simulink model "ddc_bpm_476_066_hov"  (Simulink 7.8)
settings: Solver=ode45  StartTime=0.0  StopTime=2.56e-3  RelTol=1e-3
undefined symbols (not defined in the file): dt_sim, frev_476, Fs_adc, xlipgetpartsetting
libraries: xbsIndex_r4 x654, simulink x3
(part 3 of 7)

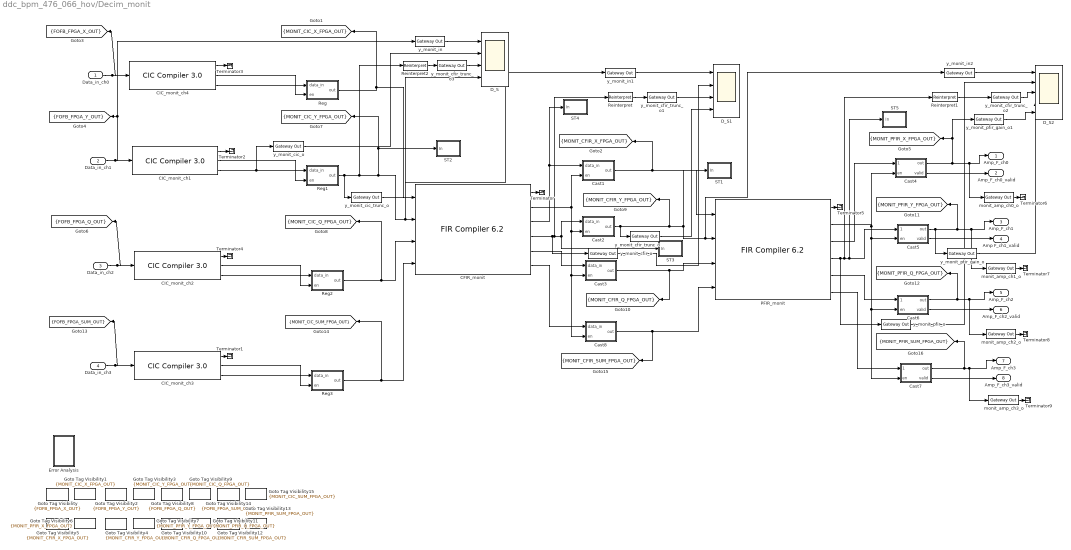
== system ddc_bpm_476_066_hov/Decim_monit ==
  Data_in_ch0 : Inport
  Data_in_ch1 : Inport  Port=2
  Data_in_ch2 : Inport  Port=3
  Data_in_ch3 : Inport  Port=4
  CFIR_monit : xbsIndex_r4/FIR Compiler 6.2   coefficientvector=hcfir_sec.Numerator  coefficient_sets=1  filter_type=Decimation  rate_change_type=Integer  interpolation_rate=1  decimation_rate=2  number_channels=1  ratespecification=Hardware_Oversampling_Rate  sampleperiod=5565000  hardwareoversamplingrate=1  filter_architecture=Systolic_Multiply_Accumulate  coefficient_reload=off  coefficient_sign=Signed  quantization=Quantize_Only  coefficient_width=16  bestprecision=on  coefficient_fractional_bits=15  coefficient_structure=Inferred  number_paths=4  output_rounding_mode=Convergent_Rounding_to_Even  output_width=25  optimization_goal=Area  data_has_tlast=Not_Required  m_data_has_tready=off  s_data_has_fifo=off  s_data_has_tuser=Not_Required  m_data_has_tuser=Not_Required  s_config_sync_mode=On_Vector  s_config_method=Single  num_reload_slots=1  has_aclken=off  has_aresetn=off  multi_column_support=Disabled  columnconfig='11'  inter_column_pipe_length=4  data_buffer_type=Automatic  coefficient_buffer_type=Automatic  input_buffer_type=Automatic  output_buffer_type=Automatic  preference_for_other_storage=Automatic  trim_axipin_name=on  passband_min=0.0  passband_max=0.5  stopband_min=0.5  stopband_max=1.0  filter_selection=1  gui_behaviour=Sysgen_GUI  data_sign=Signed  data_width=16  data_fractional_bits=0  wrapper_available=true  ip_wrap_arbitrary_binary_point=true  ip_name=FIR Compiler  ip_version=6.2  dsptool_ready=true  ipcore_usecache=true  ipcore_useipmodelcache=true  ipcore_xco_need_fpga_part=true  port_translation_map={ 'aclken' => 'en', 'aresetn' => 'rst' }  run_core_at_system_period=true  ipcore_fpga_part=xlipgetpartsetting(gcb, {'virtex6', 'xc6vlx75t', '-3', 'ff784'})  structural_sim=false  block_type=fir_compiler_v6_2
      settings: infoedit=Maximum Possible : Maximizes oversampling rate. Abstracted input handshake (no s_data_tvalid) and automatic rate propagation.<br>Hardware Oversampling Rate : Specifies oversampling rate relative to the input sample period. Abstracted input handshake (no s_data_tvalid) and automatic rate propagation.<br>Sample Period : Specifies absolute oversampling rate. No input handshake abstraction (exposes s_data_tvalid) and no rate propagation.
  CIC_monit_ch{1..4} (4 alike) : xbsIndex_r4/CIC Compiler 3.0   filter_type=Decimation  number_of_stages=5  differential_delay=2  number_of_channels=1  sample_rate_changes=Fixed  fixed_or_initial_rate=R_sec  minimum_rate=2500  maximum_rate=2500  ratespecification=Maximum_Possible  sampleperiod=1  hardwareoversamplingrate=1113  quantization=Truncation  output_data_width=25  use_xtreme_dsp_slice=off  use_streaming_interface=on  has_aclken=off  has_aresetn=off  has_dout_tready=off  trim_axipin_name=on  gui_behaviour=Sysgen_GUI  input_data_width=18  ip_name=CIC Compiler  ip_version=3.0  dsptool_ready=true  wrapper_available=true  port_translation_map={ 'aclken' => 'en', 'aresetn' => 'rst' }  ipcore_xco_need_fpga_part=true  ipcore_fpga_part=xlipgetpartsetting(gcb, {'virtex7', 'xc7v1500t', '-2', 'fhg1157'})  ipcore_verbose=false  block_type=cic_compiler_v3_0
  Cast1 : Subsystem
  Cast2 : Subsystem
  Cast3 : Subsystem
  Cast4 : Subsystem
  Cast5 : Subsystem
  Cast6 : Subsystem
  Cast7 : Subsystem
  Cast8 : Subsystem
  D_S : Scope  NumInputPorts=4
      settings: TimeRange=0.0004  YMin=0.0062~37100~0.00221125~0.0044225  YMax=0.00685~37140~0.00221375~0.0044275  MaxDataPoints=1000000  SampleInput=on
  D_S1 : Scope  NumInputPorts=4
      settings: TimeRange=0.0004  YMin=0.00442481~0.00443029~0.00443029~0.00446463  YMax=0.00442481~0.00443029~0.00443029~0.00446463  SaveName=ScopeData2  MaxDataPoints=1000000  SampleInput=on
  D_S2 : Scope  NumInputPorts=5
      settings: TimeRange=0.0004  YMin=0.00442791~-1~3.8147e-006~-3.33786e-006~-3.33786e-006  YMax=0.00442791~1~3.8147e-006~-3.33786e-006~-3.33786e-006  SaveName=ScopeData3  MaxDataPoints=1000000  SampleInput=on
  Error Analysis : Subsystem
  Goto Tag Visibility : GotoTagVisibility  GotoTag=FOFB_FPGA_X_OUT
  Goto Tag Visibility1 : GotoTagVisibility  GotoTag=MONIT_CIC_X_FPGA_OUT
  Goto Tag Visibility10 : GotoTagVisibility  GotoTag=MONIT_CFIR_Q_FPGA_OUT
  Goto Tag Visibility11 : GotoTagVisibility  GotoTag=MONIT_PFIR_Q_FPGA_OUT
  Goto Tag Visibility12 : GotoTagVisibility  GotoTag=MONIT_CFIR_SUM_FPGA_OUT
  Goto Tag Visibility13 : GotoTagVisibility  GotoTag=MONIT_PFIR_SUM_FPGA_OUT
  Goto Tag Visibility14 : GotoTagVisibility  GotoTag=FOFB_FPGA_SUM_OUT
  Goto Tag Visibility15 : GotoTagVisibility  GotoTag=MONIT_CIC_SUM_FPGA_OUT
  Goto Tag Visibility2 : GotoTagVisibility  GotoTag=FOFB_FPGA_Y_OUT
  Goto Tag Visibility3 : GotoTagVisibility  GotoTag=MONIT_CIC_Y_FPGA_OUT
  Goto Tag Visibility4 : GotoTagVisibility  GotoTag=MONIT_CFIR_Y_FPGA_OUT
  Goto Tag Visibility5 : GotoTagVisibility  GotoTag=MONIT_CFIR_X_FPGA_OUT
  Goto Tag Visibility6 : GotoTagVisibility  GotoTag=MONIT_PFIR_X_FPGA_OUT
  Goto Tag Visibility7 : GotoTagVisibility  GotoTag=MONIT_PFIR_Y_FPGA_OUT
  Goto Tag Visibility8 : GotoTagVisibility  GotoTag=FOFB_FPGA_Q_OUT
  Goto Tag Visibility9 : GotoTagVisibility  GotoTag=MONIT_CIC_Q_FPGA_OUT
  PFIR_monit : xbsIndex_r4/FIR Compiler 6.2   coefficientvector=hpfir_sec.Numerator  coefficient_sets=1  filter_type=Decimation  rate_change_type=Integer  interpolation_rate=1  decimation_rate=2  number_channels=1  ratespecification=Hardware_Oversampling_Rate  sampleperiod=5565000  hardwareoversamplingrate=1  filter_architecture=Systolic_Multiply_Accumulate  coefficient_reload=off  coefficient_sign=Signed  quantization=Quantize_Only  coefficient_width=16  bestprecision=on  coefficient_fractional_bits=15  coefficient_structure=Inferred  number_paths=4  output_rounding_mode=Convergent_Rounding_to_Even  output_width=25  optimization_goal=Area  data_has_tlast=Not_Required  m_data_has_tready=off  s_data_has_fifo=off  s_data_has_tuser=Not_Required  m_data_has_tuser=Not_Required  s_config_sync_mode=On_Vector  s_config_method=Single  num_reload_slots=1  has_aclken=off  has_aresetn=off  multi_column_support=Disabled  columnconfig='22'  inter_column_pipe_length=4  data_buffer_type=Automatic  coefficient_buffer_type=Automatic  input_buffer_type=Automatic  output_buffer_type=Automatic  preference_for_other_storage=Automatic  trim_axipin_name=on  passband_min=0.0  passband_max=0.5  stopband_min=0.5  stopband_max=1.0  filter_selection=1  gui_behaviour=Sysgen_GUI  data_sign=Signed  data_width=16  data_fractional_bits=0  wrapper_available=true  ip_wrap_arbitrary_binary_point=true  ip_name=FIR Compiler  ip_version=6.2  dsptool_ready=true  ipcore_usecache=true  ipcore_useipmodelcache=true  ipcore_xco_need_fpga_part=true  port_translation_map={ 'aclken' => 'en', 'aresetn' => 'rst' }  run_core_at_system_period=true  ipcore_fpga_part=xlipgetpartsetting(gcb, {'virtex6', 'xc6vlx75t', '-3', 'ff784'})  structural_sim=false  block_type=fir_compiler_v6_2
      settings: infoedit=Maximum Possible : Maximizes oversampling rate. Abstracted input handshake (no s_data_tvalid) and automatic rate propagation.<br>Hardware Oversampling Rate : Specifies oversampling rate relative to the input sample period. Abstracted input handshake (no s_data_tvalid) and automatic rate propagation.<br>Sample Period : Specifies absolute oversampling rate. No input handshake abstraction (exposes s_data_tvalid) and no rate propagation.
  Reg : Subsystem
  Reg1 : Subsystem
  Reg2 : Subsystem
  Reg3 : Subsystem
  Reinterpret : xbsIndex_r4/Reinterpret  force_arith_type=on  arith_type="Signed  (2's comp)"  force_bin_pt=off  bin_pt=41  block_type=cast
      settings: block_version=VER_STRING_GOES_HERE
  Reinterpret1 : xbsIndex_r4/Reinterpret  force_arith_type=on  arith_type="Signed  (2's comp)"  force_bin_pt=off  bin_pt=41  block_type=cast
      settings: block_version=VER_STRING_GOES_HERE
  Reinterpret2 : xbsIndex_r4/Reinterpret  force_arith_type=on  arith_type="Signed  (2's comp)"  force_bin_pt=on  bin_pt=23  block_type=cast
      settings: block_version=VER_STRING_GOES_HERE
  ST1 : Subsystem
  ST2 : Subsystem
  ST3 : Subsystem
  ST4 : Subsystem
  ST5 : Subsystem
  Terminator{,1..9} (10 alike) : Terminator
  monit_amp_ch0_o : xbsIndex_r4/Gateway Out  inherit_from_input=on  hdl_port=on  timing_constraint=Data Rate  locs_specified=off  LOCs={}  UseAsDAC=off  DACChannel='1'  block_type=gatewayout
      settings: infoedit="Gateway out block.  Converts Xilinx fixed-point or floating-point type inputs into ouputs of type Simulink integer, single, double, or fixed point.<br><br>Hardware notes:  In hardware these blocks become top level output ports or are discarded, depending on how they are configured."
  monit_amp_ch1_o : xbsIndex_r4/Gateway Out  inherit_from_input=on  hdl_port=on  timing_constraint=Data Rate  locs_specified=off  LOCs={}  UseAsDAC=off  DACChannel='1'  block_type=gatewayout
      settings: infoedit="Gateway out block.  Converts Xilinx fixed-point or floating-point type inputs into ouputs of type Simulink integer, single, double, or fixed point.<br><br>Hardware notes:  In hardware these blocks become top level output ports or are discarded, depending on how they are configured."
  monit_amp_ch2_o : xbsIndex_r4/Gateway Out  inherit_from_input=on  hdl_port=on  timing_constraint=Data Rate  locs_specified=off  LOCs={}  UseAsDAC=off  DACChannel='1'  block_type=gatewayout
      settings: infoedit="Gateway out block.  Converts Xilinx fixed-point or floating-point type inputs into ouputs of type Simulink integer, single, double, or fixed point.<br><br>Hardware notes:  In hardware these blocks become top level output ports or are discarded, depending on how they are configured."
  monit_amp_ch3_o : xbsIndex_r4/Gateway Out  inherit_from_input=on  hdl_port=on  timing_constraint=Data Rate  locs_specified=off  LOCs={}  UseAsDAC=off  DACChannel='1'  block_type=gatewayout
      settings: infoedit="Gateway out block.  Converts Xilinx fixed-point or floating-point type inputs into ouputs of type Simulink integer, single, double, or fixed point.<br><br>Hardware notes:  In hardware these blocks become top level output ports or are discarded, depending on how they are configured."
  y_monit_cfir_o : xbsIndex_r4/Gateway Out  inherit_from_input=on  hdl_port=off  timing_constraint=None  locs_specified=off  LOCs={}  UseAsDAC=off  DACChannel='1'  block_type=gatewayout
      settings: infoedit="Gateway out block.  Converts Xilinx fixed-point or floating-point type inputs into ouputs of type Simulink integer, single, double, or fixed point.<br><br>Hardware notes:  In hardware these blocks become top level output ports or are discarded, depending on how they are configured."
  y_monit_cfir_trunc_o{,1..3} (4 alike) : xbsIndex_r4/Gateway Out  inherit_from_input=on  hdl_port=off  timing_constraint=None  locs_specified=off  LOCs={}  UseAsDAC=off  DACChannel='1'  block_type=gatewayout
      settings: infoedit="Gateway out block.  Converts Xilinx fixed-point or floating-point type inputs into ouputs of type Simulink integer, single, double, or fixed point.<br><br>Hardware notes:  In hardware these blocks become top level output ports or are discarded, depending on how they are configured."
  y_monit_cic_o : xbsIndex_r4/Gateway Out  inherit_from_input=on  hdl_port=off  timing_constraint=None  locs_specified=off  LOCs={}  UseAsDAC=off  DACChannel='1'  block_type=gatewayout
      settings: infoedit="Gateway out block.  Converts Xilinx fixed-point or floating-point type inputs into ouputs of type Simulink integer, single, double, or fixed point.<br><br>Hardware notes:  In hardware these blocks become top level output ports or are discarded, depending on how they are configured."
  y_monit_cic_trunc_o : xbsIndex_r4/Gateway Out  inherit_from_input=on  hdl_port=off  timing_constraint=None  locs_specified=off  LOCs={}  UseAsDAC=off  DACChannel='1'  block_type=gatewayout
      settings: infoedit="Gateway out block.  Converts Xilinx fixed-point or floating-point type inputs into ouputs of type Simulink integer, single, double, or fixed point.<br><br>Hardware notes:  In hardware these blocks become top level output ports or are discarded, depending on how they are configured."
  y_monit_in : xbsIndex_r4/Gateway Out  inherit_from_input=on  hdl_port=off  timing_constraint=None  locs_specified=off  LOCs={}  UseAsDAC=off  DACChannel='1'  block_type=gatewayout
      settings: infoedit="Gateway out block.  Converts Xilinx fixed-point or floating-point type inputs into ouputs of type Simulink integer, single, double, or fixed point.<br><br>Hardware notes:  In hardware these blocks become top level output ports or are discarded, depending on how they are configured."
  y_monit_in1 : xbsIndex_r4/Gateway Out  inherit_from_input=on  hdl_port=off  timing_constraint=None  locs_specified=off  LOCs={}  UseAsDAC=off  DACChannel='1'  block_type=gatewayout
      settings: infoedit="Gateway out block.  Converts Xilinx fixed-point or floating-point type inputs into ouputs of type Simulink integer, single, double, or fixed point.<br><br>Hardware notes:  In hardware these blocks become top level output ports or are discarded, depending on how they are configured."
  y_monit_in2 : xbsIndex_r4/Gateway Out  inherit_from_input=on  hdl_port=off  timing_constraint=None  locs_specified=off  LOCs={}  UseAsDAC=off  DACChannel='1'  block_type=gatewayout
      settings: infoedit="Gateway out block.  Converts Xilinx fixed-point or floating-point type inputs into ouputs of type Simulink integer, single, double, or fixed point.<br><br>Hardware notes:  In hardware these blocks become top level output ports or are discarded, depending on how they are configured."
  y_monit_pfir_gain_o : xbsIndex_r4/Gateway Out  inherit_from_input=on  hdl_port=off  timing_constraint=None  locs_specified=off  LOCs={}  UseAsDAC=off  DACChannel='1'  block_type=gatewayout
      settings: infoedit="Gateway out block.  Converts Xilinx fixed-point or floating-point type inputs into ouputs of type Simulink integer, single, double, or fixed point.<br><br>Hardware notes:  In hardware these blocks become top level output ports or are discarded, depending on how they are configured."
  y_monit_pfir_gain_o1 : xbsIndex_r4/Gateway Out  inherit_from_input=on  hdl_port=off  timing_constraint=None  locs_specified=off  LOCs={}  UseAsDAC=off  DACChannel='1'  block_type=gatewayout
      settings: infoedit="Gateway out block.  Converts Xilinx fixed-point or floating-point type inputs into ouputs of type Simulink integer, single, double, or fixed point.<br><br>Hardware notes:  In hardware these blocks become top level output ports or are discarded, depending on how they are configured."
  y_monit_pfir_o : xbsIndex_r4/Gateway Out  inherit_from_input=on  hdl_port=off  timing_constraint=None  locs_specified=off  LOCs={}  UseAsDAC=off  DACChannel='1'  block_type=gatewayout
      settings: infoedit="Gateway out block.  Converts Xilinx fixed-point or floating-point type inputs into ouputs of type Simulink integer, single, double, or fixed point.<br><br>Hardware notes:  In hardware these blocks become top level output ports or are discarded, depending on how they are configured."
  Amp_F_ch0 : Outport
  Amp_F_ch0_valid : Outport  Port=2
  Amp_F_ch1 : Outport  Port=3
  Amp F_ch1_valid : Outport  Port=4
  Amp_F_ch2 : Outport  Port=5
  Amp_F_ch2_valid : Outport  Port=6
  Amp_F_ch3 : Outport  Port=7
  Amp_F_ch3_valid : Outport  Port=8
  tag scope: FOFB_FPGA_Q_OUT=scoped, FOFB_FPGA_SUM_OUT=scoped, FOFB_FPGA_X_OUT=scoped, FOFB_FPGA_Y_OUT=scoped, MONIT_CFIR_Q_FPGA_OUT=scoped, MONIT_CFIR_SUM_FPGA_OUT=scoped, MONIT_CFIR_X_FPGA_OUT=scoped, MONIT_CFIR_Y_FPGA_OUT=scoped, MONIT_CIC_Q_FPGA_OUT=scoped, MONIT_CIC_SUM_FPGA_OUT=scoped, MONIT_CIC_X_FPGA_OUT=scoped, MONIT_CIC_Y_FPGA_OUT=scoped, MONIT_PFIR_Q_FPGA_OUT=scoped, MONIT_PFIR_SUM_FPGA_OUT=scoped, MONIT_PFIR_X_FPGA_OUT=scoped, MONIT_PFIR_Y_FPGA_OUT=scoped
  wires:
  CIC_monit_ch4/1 -> Terminator3/1
  Cast1/1(out) -> [MONIT_CFIR_X_FPGA_OUT], PFIR_monit/1
  Reg/1(out) -> [MONIT_CIC_X_FPGA_OUT], CFIR_monit/1
  CIC_monit_ch4/3 -> Reg/1(data_in)
  Data_in_ch0/1 -> [FOFB_FPGA_X_OUT], CIC_monit_ch4/1
  CIC_monit_ch4/2 -> Reg/2(en)
  Cast4/1(out) -> Amp_F_ch0/1, monit_amp_ch0_o/1, [MONIT_PFIR_X_FPGA_OUT], y_monit_pfir_gain_o1/1
  Cast4/2(valid) -> Amp_F_ch0_valid/1
  CIC_monit_ch1/1 -> Terminator2/1
  Data_in_ch1/1 -> CIC_monit_ch1/1, [FOFB_FPGA_Y_OUT], y_monit_in/1
  Data_in_ch2/1 -> CIC_monit_ch2/1, [FOFB_FPGA_Q_OUT]
  Reg1/1(out) -> y_monit_cic_trunc_o/1, [MONIT_CIC_Y_FPGA_OUT], ST2/1(In), y_monit_in1/1, CFIR_monit/2, Reinterpret2/1
  CIC_monit_ch1/3 -> y_monit_cic_o/1, Reg1/1(data_in)
  CIC_monit_ch1/2 -> Reg1/2(en)
  Reg2/1(out) -> [MONIT_CIC_Q_FPGA_OUT], CFIR_monit/3
  CIC_monit_ch2/3 -> Reg2/1(data_in)
  CIC_monit_ch2/2 -> Reg2/2(en)
  Cast2/1(out) -> [MONIT_CFIR_Y_FPGA_OUT], ST1/1(In), y_monit_in2/1, PFIR_monit/2, y_monit_cfir_trunc_o/1
  Cast3/1(out) -> [MONIT_CFIR_Q_FPGA_OUT], PFIR_monit/3
  Cast5/1(out) -> [MONIT_PFIR_Y_FPGA_OUT], Amp_F_ch1/1, monit_amp_ch1_o/1, y_monit_pfir_gain_o/1
  Cast5/2(valid) -> Amp F_ch1_valid/1
  Cast6/1(out) -> Amp_F_ch2/1, monit_amp_ch2_o/1, [MONIT_PFIR_Q_FPGA_OUT]
  Cast6/2(valid) -> Amp_F_ch2_valid/1
  Data_in_ch3/1 -> [FOFB_FPGA_SUM_OUT], CIC_monit_ch3/1
  Reg3/1(out) -> [MONIT_CIC_SUM_FPGA_OUT], CFIR_monit/4
  CIC_monit_ch3/3 -> Reg3/1(data_in)
  CIC_monit_ch3/2 -> Reg3/2(en)
  Cast8/1(out) -> [MONIT_CFIR_SUM_FPGA_OUT], PFIR_monit/4
  CFIR_monit/6 -> Cast8/1(data_in)
  CFIR_monit/5 -> Cast3/1(data_in)
  CFIR_monit/4 -> y_monit_cfir_o/1, ST3/1(In), Cast2/1(data_in), Reinterpret/1
  CFIR_monit/3 -> ST4/1(In), Cast1/1(data_in)
  CFIR_monit/2 -> Cast3/2(en), Cast8/2(en), Cast2/2(en), Cast1/2(en)
  Cast7/1(out) -> [MONIT_PFIR_SUM_FPGA_OUT], Amp_F_ch3/1, monit_amp_ch3_o/1
  Cast7/2(valid) -> Amp_F_ch3_valid/1
  PFIR_monit/3 -> Cast4/1(data_in)
  PFIR_monit/4 -> y_monit_pfir_o/1, Reinterpret1/1, ST5/1(In), Cast5/1(data_in)
  PFIR_monit/5 -> Cast6/1(data_in)
  PFIR_monit/6 -> Cast7/1(data_in)
  PFIR_monit/2 -> Cast6/2(en), Cast7/2(en), Cast5/2(en), Cast4/2(en)
  CFIR_monit/1 -> Terminator/1
  CIC_monit_ch3/1 -> Terminator1/1
  PFIR_monit/1 -> Terminator5/1
  CIC_monit_ch2/1 -> Terminator4/1
  y_monit_cic_o/1 -> D_S/2
  y_monit_in/1 -> D_S/1
  y_monit_cfir_o/1 -> D_S1/2
  y_monit_in1/1 -> D_S1/1
  y_monit_in2/1 -> D_S2/1
  y_monit_cfir_trunc_o/1 -> D_S1/4
  Reinterpret/1 -> y_monit_cfir_trunc_o1/1
  y_monit_cfir_trunc_o1/1 -> D_S1/3
  y_monit_pfir_o/1 -> D_S2/2
  y_monit_pfir_gain_o/1 -> D_S2/4
  Reinterpret1/1 -> y_monit_cfir_trunc_o2/1
  y_monit_cfir_trunc_o2/1 -> D_S2/3
  y_monit_cic_trunc_o/1 -> D_S/4
  Reinterpret2/1 -> y_monit_cfir_trunc_o3/1
  y_monit_cfir_trunc_o3/1 -> D_S/3
  monit_amp_ch0_o/1 -> Terminator6/1
  monit_amp_ch1_o/1 -> Terminator7/1
  monit_amp_ch2_o/1 -> Terminator8/1
  monit_amp_ch3_o/1 -> Terminator9/1
  y_monit_pfir_gain_o1/1 -> D_S2/5

== system ddc_bpm_476_066_hov/Ksum_fofb_mult ==
  In1 : Inport
  In2 : Inport  Port=2
  Cast_truncate1 : Subsystem
  Kx_tbt : xbsIndex_r4/Mult  precision=Full  arith_type="Signed  (2's comp)"  n_bits=16  bin_pt=14  quantization=Truncate  overflow=Wrap  en=off  latency=8  dbl_ovrd=off  use_behavioral_HDL=off  opt=Speed  use_embedded=off  optimum_pipeline=on  pipeline=on  use_rpm=on  placement_style=Triangular  block_type=mult
  Out1 : Outport
  wires:
  Kx_tbt/1 -> Cast_truncate1/1(In1)
  In1/1 -> Kx_tbt/1
  Cast_truncate1/1(Out1) -> Out1/1
  In2/1 -> Kx_tbt/2

== system ddc_bpm_476_066_hov/Ksum_tbt_mult2 ==
  In1 : Inport
  In2 : Inport  Port=2
  Cast_truncate1 : Subsystem
  Kx_tbt : xbsIndex_r4/Mult  precision=Full  arith_type="Signed  (2's comp)"  n_bits=16  bin_pt=14  quantization=Truncate  overflow=Wrap  en=off  latency=8  dbl_ovrd=off  use_behavioral_HDL=off  opt=Speed  use_embedded=off  optimum_pipeline=on  pipeline=on  use_rpm=on  placement_style=Triangular  block_type=mult
  Out1 : Outport
  wires:
  Kx_tbt/1 -> Cast_truncate1/1(In1)
  In1/1 -> Kx_tbt/1
  Cast_truncate1/1(Out1) -> Out1/1
  In2/1 -> Kx_tbt/2

== system ddc_bpm_476_066_hov/Ksum_tbt_mult3 ==
  In1 : Inport
  In2 : Inport  Port=2
  Cast_truncate1 : Subsystem
  Kx_tbt : xbsIndex_r4/Mult  precision=Full  arith_type="Signed  (2's comp)"  n_bits=16  bin_pt=14  quantization=Truncate  overflow=Wrap  en=off  latency=8  dbl_ovrd=off  use_behavioral_HDL=off  opt=Speed  use_embedded=off  optimum_pipeline=on  pipeline=on  use_rpm=on  placement_style=Triangular  block_type=mult
  Out1 : Outport
  wires:
  Kx_tbt/1 -> Cast_truncate1/1(In1)
  In1/1 -> Kx_tbt/1
  Cast_truncate1/1(Out1) -> Out1/1
  In2/1 -> Kx_tbt/2

== system ddc_bpm_476_066_hov/Kx_fofb_mult ==
  In1 : Inport
  In2 : Inport  Port=2
  Cast_truncate1 : Subsystem
  Kx_tbt : xbsIndex_r4/Mult  precision=Full  arith_type="Signed  (2's comp)"  n_bits=16  bin_pt=14  quantization=Truncate  overflow=Wrap  en=off  latency=8  dbl_ovrd=off  use_behavioral_HDL=off  opt=Speed  use_embedded=off  optimum_pipeline=on  pipeline=on  use_rpm=on  placement_style=Triangular  block_type=mult
  Out1 : Outport
  wires:
  Kx_tbt/1 -> Cast_truncate1/1(In1)
  In1/1 -> Kx_tbt/1
  Cast_truncate1/1(Out1) -> Out1/1
  In2/1 -> Kx_tbt/2

== system ddc_bpm_476_066_hov/Kx_monit_mult ==
  In1 : Inport
  In2 : Inport  Port=2
  Cast_truncate1 : Subsystem
  Kx_tbt : xbsIndex_r4/Mult  precision=Full  arith_type="Signed  (2's comp)"  n_bits=16  bin_pt=14  quantization=Truncate  overflow=Wrap  en=off  latency=8  dbl_ovrd=off  use_behavioral_HDL=off  opt=Speed  use_embedded=off  optimum_pipeline=on  pipeline=on  use_rpm=on  placement_style=Triangular  block_type=mult
  Out1 : Outport
  wires:
  Kx_tbt/1 -> Cast_truncate1/1(In1)
  In1/1 -> Kx_tbt/1
  Cast_truncate1/1(Out1) -> Out1/1
  In2/1 -> Kx_tbt/2

== system ddc_bpm_476_066_hov/Kx_q_fofb_mult ==
  In1 : Inport
  In2 : Inport  Port=2
  Cast_truncate1 : Subsystem
  Kx_tbt : xbsIndex_r4/Mult  precision=Full  arith_type="Signed  (2's comp)"  n_bits=16  bin_pt=14  quantization=Truncate  overflow=Wrap  en=off  latency=8  dbl_ovrd=off  use_behavioral_HDL=off  opt=Speed  use_embedded=off  optimum_pipeline=on  pipeline=on  use_rpm=on  placement_style=Triangular  block_type=mult
  Out1 : Outport
  wires:
  Kx_tbt/1 -> Cast_truncate1/1(In1)
  In1/1 -> Kx_tbt/1
  Cast_truncate1/1(Out1) -> Out1/1
  In2/1 -> Kx_tbt/2

== system ddc_bpm_476_066_hov/Kx_q_monit_mult ==
  In1 : Inport
  In2 : Inport  Port=2
  Cast_truncate1 : Subsystem
  Kx_tbt : xbsIndex_r4/Mult  precision=Full  arith_type="Signed  (2's comp)"  n_bits=16  bin_pt=14  quantization=Truncate  overflow=Wrap  en=off  latency=8  dbl_ovrd=off  use_behavioral_HDL=off  opt=Speed  use_embedded=off  optimum_pipeline=on  pipeline=on  use_rpm=on  placement_style=Triangular  block_type=mult
  Out1 : Outport
  wires:
  Kx_tbt/1 -> Cast_truncate1/1(In1)
  In1/1 -> Kx_tbt/1
  Cast_truncate1/1(Out1) -> Out1/1
  In2/1 -> Kx_tbt/2

== system ddc_bpm_476_066_hov/Kx_q_tbt_mult ==
  In1 : Inport
  In2 : Inport  Port=2
  Cast_truncate1 : Subsystem
  Kx_tbt : xbsIndex_r4/Mult  precision=Full  arith_type="Signed  (2's comp)"  n_bits=16  bin_pt=14  quantization=Truncate  overflow=Wrap  en=off  latency=8  dbl_ovrd=off  use_behavioral_HDL=off  opt=Speed  use_embedded=off  optimum_pipeline=on  pipeline=on  use_rpm=on  placement_style=Triangular  block_type=mult
  Out1 : Outport
  wires:
  Kx_tbt/1 -> Cast_truncate1/1(In1)
  In1/1 -> Kx_tbt/1
  Cast_truncate1/1(Out1) -> Out1/1
  In2/1 -> Kx_tbt/2

== system ddc_bpm_476_066_hov/Kx_tbt_mult ==
  In1 : Inport
  In2 : Inport  Port=2
  Cast_truncate1 : Subsystem
  Kx_tbt : xbsIndex_r4/Mult  precision=Full  arith_type="Signed  (2's comp)"  n_bits=16  bin_pt=14  quantization=Truncate  overflow=Wrap  en=off  latency=8  dbl_ovrd=off  use_behavioral_HDL=off  opt=Speed  use_embedded=off  optimum_pipeline=on  pipeline=on  use_rpm=on  placement_style=Triangular  block_type=mult
  Out1 : Outport
  wires:
  Kx_tbt/1 -> Cast_truncate1/1(In1)
  In1/1 -> Kx_tbt/1
  Cast_truncate1/1(Out1) -> Out1/1
  In2/1 -> Kx_tbt/2

== system ddc_bpm_476_066_hov/Ky_fofb_mult ==
  In1 : Inport
  In2 : Inport  Port=2
  Cast_truncate1 : Subsystem
  Kx_tbt : xbsIndex_r4/Mult  precision=Full  arith_type="Signed  (2's comp)"  n_bits=16  bin_pt=14  quantization=Truncate  overflow=Wrap  en=off  latency=8  dbl_ovrd=off  use_behavioral_HDL=off  opt=Speed  use_embedded=off  optimum_pipeline=on  pipeline=on  use_rpm=on  placement_style=Triangular  block_type=mult
  Out1 : Outport
  wires:
  Kx_tbt/1 -> Cast_truncate1/1(In1)
  In1/1 -> Kx_tbt/1
  Cast_truncate1/1(Out1) -> Out1/1
  In2/1 -> Kx_tbt/2

== system ddc_bpm_476_066_hov/Ky_monit_mult ==
  In1 : Inport
  In2 : Inport  Port=2
  Cast_truncate1 : Subsystem
  Kx_tbt : xbsIndex_r4/Mult  precision=Full  arith_type="Signed  (2's comp)"  n_bits=16  bin_pt=14  quantization=Truncate  overflow=Wrap  en=off  latency=8  dbl_ovrd=off  use_behavioral_HDL=off  opt=Speed  use_embedded=off  optimum_pipeline=on  pipeline=on  use_rpm=on  placement_style=Triangular  block_type=mult
  Out1 : Outport
  wires:
  Kx_tbt/1 -> Cast_truncate1/1(In1)
  In1/1 -> Kx_tbt/1
  Cast_truncate1/1(Out1) -> Out1/1
  In2/1 -> Kx_tbt/2

== system ddc_bpm_476_066_hov/Ky_tbt_mult ==
  In1 : Inport
  In2 : Inport  Port=2
  Cast_truncate1 : Subsystem
  Kx_tbt : xbsIndex_r4/Mult  precision=Full  arith_type="Signed  (2's comp)"  n_bits=16  bin_pt=14  quantization=Truncate  overflow=Wrap  en=off  latency=8  dbl_ovrd=off  use_behavioral_HDL=off  opt=Speed  use_embedded=off  optimum_pipeline=on  pipeline=on  use_rpm=on  placement_style=Triangular  block_type=mult
  Out1 : Outport
  wires:
  Kx_tbt/1 -> Cast_truncate1/1(In1)
  In1/1 -> Kx_tbt/1
  Cast_truncate1/1(Out1) -> Out1/1
  In2/1 -> Kx_tbt/2

== system ddc_bpm_476_066_hov/debug_analysis ==
  Constant : Constant  Value=0
  D_S2 : Scope  NumInputPorts=6
      settings: TimeRange=0.0004  YMin=-1~434.15~10~-5~-1.5~-1.5  YMax=1~479.85~100~5~1.5~1.5  SaveName=ScopeData8  MaxDataPoints=1000000  SampleInput=on
  D_S3 : Scope  NumInputPorts=4
      settings: TimeRange=0.0004  YMin=-1~-1.5~10~-1.5  YMax=1~1.5~100~1.5  SaveName=ScopeData9  MaxDataPoints=1000000  SampleInput=on
  D_S4 : Scope  NumInputPorts=4
      settings: TimeRange=0.0004  YMin=0.95~0.95~10~-1.5  YMax=1.05~1.05~100~1.5  SaveName=ScopeData10  MaxDataPoints=1000000  SampleInput=on
  q_tbt_o2 : xbsIndex_r4/Gateway Out  inherit_from_input=on  hdl_port=off  timing_constraint=None  locs_specified=off  LOCs={}  UseAsDAC=off  DACChannel='1'  block_type=gatewayout
      settings: infoedit="Gateway out block.  Converts Xilinx fixed-point or floating-point type inputs into ouputs of type Simulink integer, single, double, or fixed point.<br><br>Hardware notes:  In hardware these blocks become top level output ports or are discarded, depending on how they are configured."
  q_tbt_o3 : xbsIndex_r4/Gateway Out  inherit_from_input=on  hdl_port=off  timing_constraint=None  locs_specified=off  LOCs={}  UseAsDAC=off  DACChannel='1'  block_type=gatewayout
      settings: infoedit="Gateway out block.  Converts Xilinx fixed-point or floating-point type inputs into ouputs of type Simulink integer, single, double, or fixed point.<br><br>Hardware notes:  In hardware these blocks become top level output ports or are discarded, depending on how they are configured."
  sum_tbt_o2 : xbsIndex_r4/Gateway Out  inherit_from_input=on  hdl_port=off  timing_constraint=None  locs_specified=off  LOCs={}  UseAsDAC=off  DACChannel='1'  block_type=gatewayout
      settings: infoedit="Gateway out block.  Converts Xilinx fixed-point or floating-point type inputs into ouputs of type Simulink integer, single, double, or fixed point.<br><br>Hardware notes:  In hardware these blocks become top level output ports or are discarded, depending on how they are configured."
  sum_tbt_o3 : xbsIndex_r4/Gateway Out  inherit_from_input=on  hdl_port=off  timing_constraint=None  locs_specified=off  LOCs={}  UseAsDAC=off  DACChannel='1'  block_type=gatewayout
      settings: infoedit="Gateway out block.  Converts Xilinx fixed-point or floating-point type inputs into ouputs of type Simulink integer, single, double, or fixed point.<br><br>Hardware notes:  In hardware these blocks become top level output ports or are discarded, depending on how they are configured."
  x_tbt_o{2..5} (4 alike) : xbsIndex_r4/Gateway Out  inherit_from_input=on  hdl_port=off  timing_constraint=None  locs_specified=off  LOCs={}  UseAsDAC=off  DACChannel='1'  block_type=gatewayout
      settings: infoedit="Gateway out block.  Converts Xilinx fixed-point or floating-point type inputs into ouputs of type Simulink integer, single, double, or fixed point.<br><br>Hardware notes:  In hardware these blocks become top level output ports or are discarded, depending on how they are configured."
  y_tbt_o{2..5,7} (5 alike) : xbsIndex_r4/Gateway Out  inherit_from_input=on  hdl_port=off  timing_constraint=None  locs_specified=off  LOCs={}  UseAsDAC=off  DACChannel='1'  block_type=gatewayout
      settings: infoedit="Gateway out block.  Converts Xilinx fixed-point or floating-point type inputs into ouputs of type Simulink integer, single, double, or fixed point.<br><br>Hardware notes:  In hardware these blocks become top level output ports or are discarded, depending on how they are configured."
  wires:
  [DELTA_X_D_S_FPGA_VALID] -> x_tbt_o2/1
  [DELTA_SUM_D_S_FPGA_VALID] -> sum_tbt_o2/1
  [DELTA_Y_D_S_FPGA_VALID] -> y_tbt_o2/1
  [DELTA_Q_D_S_FPGA_VALID] -> q_tbt_o2/1
  x_tbt_o2/1 -> D_S2/1
  y_tbt_o2/1 -> D_S2/2
  q_tbt_o2/1 -> D_S2/3
  sum_tbt_o2/1 -> D_S2/4
  [Y_DIVIDOR_D_S_FPGA_RDY] -> sum_tbt_o3/1
  [Y_DIVIDEND_D_S_FPGA_RDY] -> q_tbt_o3/1
  q_tbt_o3/1 -> D_S2/5
  sum_tbt_o3/1 -> D_S2/6
  [Y_DIVIDEND_D_S_FPGA] -> x_tbt_o3/1
  [Y_DIVIDEND_D_S_FPGA_VALID] -> y_tbt_o3/1
  x_tbt_o3/1 -> D_S3/1
  y_tbt_o3/1 -> D_S3/2
  [SUM_DIVISOR_D_S_FPGA] -> x_tbt_o4/1
  [SUM_DIVISOR_D_S_FPGA_VALID] -> y_tbt_o4/1
  x_tbt_o4/1 -> D_S3/3
  y_tbt_o4/1 -> D_S3/4
  [D_S_FPGA_CE_DOUTY] -> x_tbt_o5/1
  [D_S_FPGA_CE_FRACY] -> y_tbt_o5/1
  x_tbt_o5/1 -> D_S4/1
  y_tbt_o5/1 -> D_S4/2
  [D_S_FPGA_Y_DIVIDER_QUOC] -> y_tbt_o7/1
  y_tbt_o7/1 -> D_S4/3
  Constant/1 -> D_S4/4

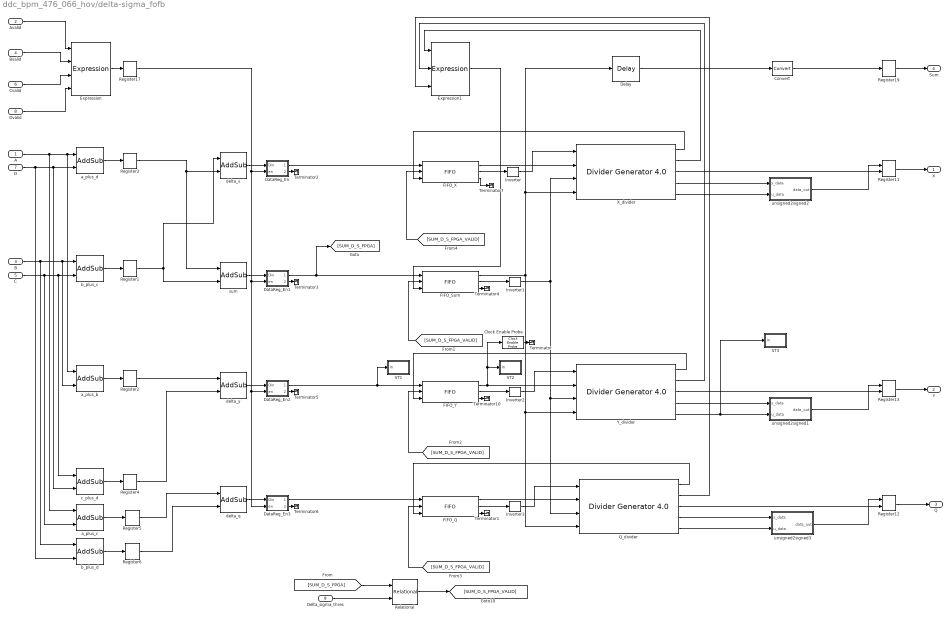
== system ddc_bpm_476_066_hov/delta-sigma_fofb ==
  A : Inport
  Avalid : Inport  Port=2
  B : Inport  Port=3
  Bvalid : Inport  Port=4
  C : Inport  Port=5
  Cvalid : Inport  Port=6
  D : Inport  Port=7
  Dvalid : Inport  Port=8
  Delta_sigma_thres : Inport  Port=9
  Clock Enable Probe : xbsIndex_r4/Clock Enable Probe  inherit_constraints=on  block_type=ceprobe
      settings: infoedit="Clock enable extractor.  Produces a Boolean output that mirrors the hardware clock enable associated with the input sample rate.<br><br>Hardware notes: in hardware this block costs nothing."
  Convert : xbsIndex_r4/Convert  gui_display_data_type=Fixed-point  arith_type="Signed  (2's comp)"  n_bits=24  bin_pt=20  float_type=Single  exp_bits=8  fraction_bits=24  quantization="Round  (unbiased: +/- Inf)"  overflow=Flag as error  en=off  latency=0  dbl_ovrd=off  pipeline=off  block_type=convert
  DataReg_En : Subsystem
  DataReg_En1 : Subsystem
  DataReg_En2 : Subsystem
  DataReg_En3 : Subsystem
  Delay : xbsIndex_r4/Delay  rst=off  infoeditControl=Selection of Reset will increase slice count due to use of real FFs and instead of SRLs  en=off  latency=25  dbl_ovrd=off  reg_retiming=off  block_type=delay
  Expression : xbsIndex_r4/Expression  expression=a & b & c & d  align_bp=on  en=off  latency=0  precision=Full  arith_type=Unsigned  n_bits=16  bin_pt=0  dbl_ovrd=off  block_type=expr
  Expression1 : xbsIndex_r4/Expression  expression=a & b & c  align_bp=on  en=off  latency=0  precision=Full  arith_type=Unsigned  n_bits=16  bin_pt=0  dbl_ovrd=off  block_type=expr
  FIFO_Q : xbsIndex_r4/FIFO  performance_options=First_Word_Fall_Through  depth=16  percent_nbits=1  rst=off  en=off  use_dcount=off  use_percent_full_port=off  use_almost_empty=off  almost_empty_thresh=2  use_almost_full=off  almost_full_thresh=14  dbl_ovrd=off  mem_type=Distributed RAM  explicit_period=off  block_type=fifo
  FIFO_Sum : xbsIndex_r4/FIFO  performance_options=First_Word_Fall_Through  depth=16  percent_nbits=1  rst=off  en=off  use_dcount=off  use_percent_full_port=off  use_almost_empty=off  almost_empty_thresh=2  use_almost_full=off  almost_full_thresh=14  dbl_ovrd=off  mem_type=Distributed RAM  explicit_period=off  block_type=fifo
  FIFO_X : xbsIndex_r4/FIFO  performance_options=First_Word_Fall_Through  depth=16  percent_nbits=1  rst=off  en=off  use_dcount=off  use_percent_full_port=off  use_almost_empty=off  almost_empty_thresh=2  use_almost_full=off  almost_full_thresh=14  dbl_ovrd=off  mem_type=Distributed RAM  explicit_period=off  block_type=fifo
  FIFO_Y : xbsIndex_r4/FIFO  performance_options=First_Word_Fall_Through  depth=16  percent_nbits=1  rst=off  en=off  use_dcount=off  use_percent_full_port=off  use_almost_empty=off  almost_empty_thresh=2  use_almost_full=off  almost_full_thresh=14  dbl_ovrd=off  mem_type=Distributed RAM  explicit_period=off  block_type=fifo
  Inverter{,1..3} (4 alike) : xbsIndex_r4/Inverter  en=off  latency=0  dbl_ovrd=off  block_type=inv
  Q_divider : xbsIndex_r4/Divider Generator 4.0   algorithm_type=High_Radix  remainder_type=Fractional  fractional_width=23  clocks_per_division=1  divide_by_zero_detect=off  flowcontrol=NonBlocking  optimizegoal=Performance  latency_configuration=Manual  latency=25  dividend_has_tuser=off  dividend_has_tlast=off  divisor_has_tuser=off  divisor_has_tlast=off  aclken=off  aresetn=off  outtready=off  outtlastbehv=Null  trim_axipin_name=on  dividend_tuser_width=1  divisor_tuser_width=1  operand_sign=Signed  dividend_and_quotient_width=16  divisor_width=16  ip_name=Divider Generator  ip_version=4.0  dsptool_ready=true  ipcore_usecache=true  ipcore_useipmodelcache=true  wrapper_available=true  port_translation_map={'aclken' => 'en','aresetn' => 'rst'}  ipcore_fpga_part=xlipgetpartsetting(gcb, {'virtex7', 'xc7v1500t', '-2', 'fhg1157'})  ipcore_verbose=false  block_type=div_gen_v4_0
      settings: infoedit=Divider Generator 4.0
  Register{1..6,17,19} (8 alike) : xbsIndex_r4/Register  init=0  rst=off  en=off  dbl_ovrd=off  block_type=register
  Register11 : xbsIndex_r4/Register  init=0  rst=off  en=on  dbl_ovrd=off  block_type=register
  Register12 : xbsIndex_r4/Register  init=0  rst=off  en=on  dbl_ovrd=off  block_type=register
  Register13 : xbsIndex_r4/Register  init=0  rst=off  en=on  dbl_ovrd=off  block_type=register
  Relational : xbsIndex_r4/Relational  mode=a>b  en=off  latency=0  dbl_ovrd=off  block_type=relational
  ST1 : Subsystem
  ST2 : Subsystem
  ST3 : Subsystem
  Terminator{,1..7,10} (9 alike) : Terminator
  X_divider : xbsIndex_r4/Divider Generator 4.0   algorithm_type=High_Radix  remainder_type=Fractional  fractional_width=23  clocks_per_division=1  divide_by_zero_detect=off  flowcontrol=NonBlocking  optimizegoal=Performance  latency_configuration=Manual  latency=25  dividend_has_tuser=off  dividend_has_tlast=off  divisor_has_tuser=off  divisor_has_tlast=off  aclken=off  aresetn=off  outtready=off  outtlastbehv=Null  trim_axipin_name=on  dividend_tuser_width=1  divisor_tuser_width=1  operand_sign=Signed  dividend_and_quotient_width=16  divisor_width=16  ip_name=Divider Generator  ip_version=4.0  dsptool_ready=true  ipcore_usecache=true  ipcore_useipmodelcache=true  wrapper_available=true  port_translation_map={'aclken' => 'en','aresetn' => 'rst'}  ipcore_fpga_part=xlipgetpartsetting(gcb, {'virtex7', 'xc7v1500t', '-2', 'fhg1157'})  ipcore_verbose=false  block_type=div_gen_v4_0
      settings: infoedit=Divider Generator 4.0
  Y_divider : xbsIndex_r4/Divider Generator 4.0   algorithm_type=High_Radix  remainder_type=Fractional  fractional_width=23  clocks_per_division=1  divide_by_zero_detect=off  flowcontrol=NonBlocking  optimizegoal=Performance  latency_configuration=Manual  latency=25  dividend_has_tuser=off  dividend_has_tlast=off  divisor_has_tuser=off  divisor_has_tlast=off  aclken=off  aresetn=off  outtready=off  outtlastbehv=Null  trim_axipin_name=on  dividend_tuser_width=1  divisor_tuser_width=1  operand_sign=Signed  dividend_and_quotient_width=16  divisor_width=16  ip_name=Divider Generator  ip_version=4.0  dsptool_ready=true  ipcore_usecache=true  ipcore_useipmodelcache=true  wrapper_available=true  port_translation_map={'aclken' => 'en','aresetn' => 'rst'}  ipcore_fpga_part=xlipgetpartsetting(gcb, {'virtex7', 'xc7v1500t', '-2', 'fhg1157'})  ipcore_verbose=false  block_type=div_gen_v4_0
      settings: infoedit=Divider Generator 4.0
  a_plus_b : xbsIndex_r4/AddSub  mode=Addition  use_carryin=off  use_carryout=off  en=off  latency=0  precision=Full  arith_type=Unsigned  n_bits=16  bin_pt=14  quantization=Truncate  overflow=Wrap  dbl_ovrd=off  use_behavioral_HDL=off  hw_selection=Fabric  pipelined=off  block_type=addsub
  a_plus_c : xbsIndex_r4/AddSub  mode=Addition  use_carryin=off  use_carryout=off  en=off  latency=0  precision=Full  arith_type=Unsigned  n_bits=16  bin_pt=14  quantization=Truncate  overflow=Wrap  dbl_ovrd=off  use_behavioral_HDL=off  hw_selection=Fabric  pipelined=off  block_type=addsub
  a_plus_d : xbsIndex_r4/AddSub  mode=Addition  use_carryin=off  use_carryout=off  en=off  latency=0  precision=Full  arith_type=Unsigned  n_bits=16  bin_pt=14  quantization=Truncate  overflow=Wrap  dbl_ovrd=off  use_behavioral_HDL=off  hw_selection=Fabric  pipelined=off  block_type=addsub
  b_plus_c : xbsIndex_r4/AddSub  mode=Addition  use_carryin=off  use_carryout=off  en=off  latency=0  precision=Full  arith_type=Unsigned  n_bits=16  bin_pt=14  quantization=Truncate  overflow=Wrap  dbl_ovrd=off  use_behavioral_HDL=off  hw_selection=Fabric  pipelined=off  block_type=addsub
  b_plus_d : xbsIndex_r4/AddSub  mode=Addition  use_carryin=off  use_carryout=off  en=off  latency=0  precision=Full  arith_type=Unsigned  n_bits=16  bin_pt=14  quantization=Truncate  overflow=Wrap  dbl_ovrd=off  use_behavioral_HDL=off  hw_selection=Fabric  pipelined=off  block_type=addsub
  c_plus_d : xbsIndex_r4/AddSub  mode=Addition  use_carryin=off  use_carryout=off  en=off  latency=0  precision=Full  arith_type=Unsigned  n_bits=16  bin_pt=14  quantization=Truncate  overflow=Wrap  dbl_ovrd=off  use_behavioral_HDL=off  hw_selection=Fabric  pipelined=off  block_type=addsub
  delta_q : xbsIndex_r4/AddSub  mode=Subtraction  use_carryin=off  use_carryout=off  en=off  latency=0  precision=Full  arith_type=Unsigned  n_bits=16  bin_pt=14  quantization=Truncate  overflow=Wrap  dbl_ovrd=off  use_behavioral_HDL=off  hw_selection=Fabric  pipelined=off  block_type=addsub
  delta_x : xbsIndex_r4/AddSub  mode=Subtraction  use_carryin=off  use_carryout=off  en=off  latency=0  precision=Full  arith_type=Unsigned  n_bits=16  bin_pt=14  quantization=Truncate  overflow=Wrap  dbl_ovrd=off  use_behavioral_HDL=off  hw_selection=Fabric  pipelined=off  block_type=addsub
  delta_y : xbsIndex_r4/AddSub  mode=Subtraction  use_carryin=off  use_carryout=off  en=off  latency=0  precision=Full  arith_type=Unsigned  n_bits=16  bin_pt=14  quantization=Truncate  overflow=Wrap  dbl_ovrd=off  use_behavioral_HDL=off  hw_selection=Fabric  pipelined=off  block_type=addsub
  sum : xbsIndex_r4/AddSub  mode=Addition  use_carryin=off  use_carryout=off  en=off  latency=0  precision=Full  arith_type=Unsigned  n_bits=16  bin_pt=14  quantization=Truncate  overflow=Wrap  dbl_ovrd=off  use_behavioral_HDL=off  hw_selection=Fabric  pipelined=off  block_type=addsub
  unsigned2signed1 : Subsystem
  unsigned2signed2 : Subsystem
  unsigned2signed3 : Subsystem
  X : Outport
  Y : Outport  Port=2
  Q : Outport  Port=3
  Sum : Outport  Port=4
  wires:
  A/1 -> a_plus_d/1, a_plus_b/1, a_plus_c/1
  D/1 -> a_plus_d/2, c_plus_d/2, b_plus_d/2
  B/1 -> b_plus_c/1, a_plus_b/2, b_plus_d/1
  C/1 -> b_plus_c/2, c_plus_d/1, a_plus_c/2
  a_plus_d/1 -> Register3/1
  b_plus_c/1 -> Register1/1
  a_plus_b/1 -> Register2/1
  c_plus_d/1 -> Register4/1
  a_plus_c/1 -> Register5/1
  b_plus_d/1 -> Register6/1
  Register3/1 -> sum/1, delta_x/2
  Register1/1 -> sum/2, delta_x/1
  Register2/1 -> delta_y/1
  Register4/1 -> delta_y/2
  Register5/1 -> delta_q/1
  Register6/1 -> delta_q/2
  delta_q/1 -> DataReg_En3/1(Din)
  delta_x/1 -> DataReg_En/1(Din)
  Register19/1 -> Sum/1
  Avalid/1 -> Expression/1
  Bvalid/1 -> Expression/2
  Cvalid/1 -> Expression/3
  Dvalid/1 -> Expression/4
  Expression/1 -> Register17/1
  DataReg_En1/1(Dout) -> FIFO_Sum/1, [SUM_D_S_FPGA]
  Register17/1 -> DataReg_En/2(en), DataReg_En1/2(en), DataReg_En2/2(en), DataReg_En3/2(en)
  Register13/1 -> Y/1
  Register11/1 -> X/1
  Register12/1 -> Q/1
  sum/1 -> DataReg_En1/1(Din)
  delta_y/1 -> DataReg_En2/1(Din)
  Delay/1 -> Convert/1
  X_divider/3 -> Register11/2
  DataReg_En/1(Dout) -> FIFO_X/1
  Y_divider/5 -> unsigned2signed1/2(u_data), ST3/1(In)
  Y_divider/3 -> Register13/2
  Q_divider/3 -> Register12/2
  DataReg_En2/1(Dout) -> FIFO_Y/1, ST1/1(In)
  DataReg_En3/1(Dout) -> FIFO_Q/1
  X_divider/2 -> Expression1/1
  Y_divider/1 -> FIFO_Y/3
  Y_divider/2 -> Expression1/2
  Delta_sigma_thres/1 -> Relational/2
  [SUM_D_S_FPGA] -> Relational/1
  Relational/1 -> [SUM_D_S_FPGA_VALID]
  [SUM_D_S_FPGA_VALID] -> FIFO_Sum/2
  FIFO_Sum/1 -> Y_divider/4, Q_divider/4, X_divider/4, Delay/1
  FIFO_X/1 -> X_divider/2
  FIFO_Q/1 -> Q_divider/2
  FIFO_Y/1 -> ST2/1(In), Clock Enable Probe/1, Y_divider/2
  Q_divider/2 -> Expression1/3
  Expression1/1 -> FIFO_Sum/3
  X_divider/1 -> FIFO_X/3
  Q_divider/1 -> FIFO_Q/3
  [SUM_D_S_FPGA_VALID] -> FIFO_Y/2
  [SUM_D_S_FPGA_VALID] -> FIFO_Q/2
  FIFO_Q/2 -> Inverter3/1
  FIFO_Q/3 -> Terminator1/1
  FIFO_Sum/2 -> Inverter1/1
  FIFO_Sum/3 -> Terminator4/1
  FIFO_X/3 -> Terminator7/1
  FIFO_Y/2 -> Inverter2/1
  FIFO_Y/3 -> Terminator10/1
  [SUM_D_S_FPGA_VALID] -> FIFO_X/2
  FIFO_X/2 -> Inverter/1
  Inverter/1 -> X_divider/1
  Inverter1/1 -> Y_divider/3, Q_divider/3, X_divider/3
  Inverter2/1 -> Y_divider/1
  Inverter3/1 -> Q_divider/1
  X_divider/5 -> unsigned2signed2/2(u_data)
  X_divider/4 -> unsigned2signed2/1(s_data)
  unsigned2signed2/1(data_out) -> Register11/1
  Y_divider/4 -> unsigned2signed1/1(s_data)
  unsigned2signed1/1(data_out) -> Register13/1
  Q_divider/5 -> unsigned2signed3/2(u_data)
  Q_divider/4 -> unsigned2signed3/1(s_data)
  unsigned2signed3/1(data_out) -> Register12/1
  Clock Enable Probe/1 -> Terminator/1
  DataReg_En/2(Valid) -> Terminator2/1
  DataReg_En1/2(Valid) -> Terminator3/1
  DataReg_En2/2(Valid) -> Terminator5/1
  DataReg_En3/2(Valid) -> Terminator6/1
  Convert/1 -> Register19/1
